simulink model "Snake_Robot_Head_Control"  (R2023a)
settings: Solver=ode23tb  StartTime=0.0  StopTime=2000  FixedStep=0.001  RelTol=1e-3
values from neighbouring files (symbols this model uses):
  cn = 5    [parameters_Robot_control.m]
  ct = 1    [parameters_Robot_control.m]
undefined symbols (not defined in the file or in its folder): X, Y, Z
libraries: nesl_utility x85, sm_lib x49
(part 1 of 3)
settings Model: PacingRate=0.100000  Creator=Bhavik  LastModifiedBy=Bhavik
settings SolverCC: ZeroCrossAlgorithm=Adaptive
settings OptimizationCC: ReuseModelBlockBuffer=off
settings DebuggingCC: UnconnectedInputMsg=warning  UnconnectedOutputMsg=warning  UnconnectedLineMsg=warning
settings ModelReferenceCC: EnableRefExpFcnMdlSchedulingChecks=on
settings RTWCC: DLArmComputeVersion=19.05

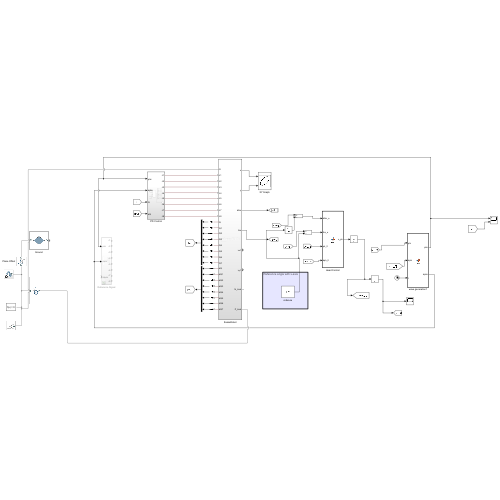
[thumbnail: Simulink's stored preview of the top-level diagram]
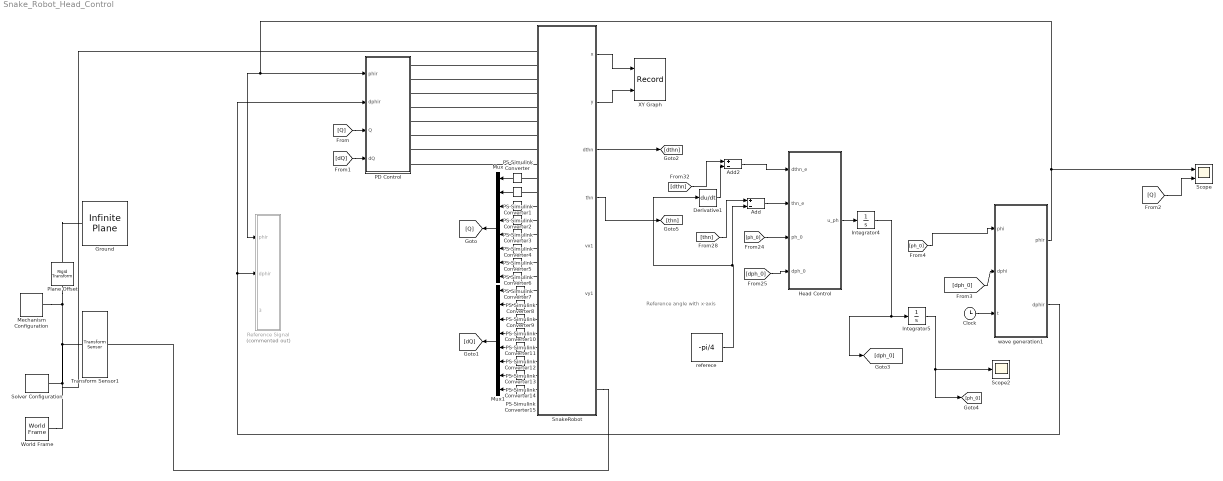
== system Snake_Robot_Head_Control ==
  note: Reference angle with x-axis
  Add : Sum  Inputs=+-
  Add2 : Sum  Inputs=+-
  Clock : Clock
  Derivative1 : Derivative
  Ground : sm_lib/Curves and Surfaces/Infinite Plane  GraphicType=Rectangle  GraphicPlaneWidth=900  GraphicPlaneWidthUnits=m  GraphicPlaneHeight=900  GraphicPlaneHeightUnits=m  GraphicVisPropType=AdvancedVisualProperties  GraphicDiffuseColor=[1 1 1]  GraphicOpacity=1  GraphicSpecularColor=[1 0.4118 0.1608]  GraphicAmbientColor=[0.302 0.7451 0.9333]  GraphicEmissiveColor=[0 1 1]  GraphicShininess=75
  Head Control : MATLAB Function  TreatAsAtomicUnit=on
  Integrator4 : Integrator
  Integrator5 : Integrator
  Mechanism Configuration : sm_lib/Utilities/Mechanism Configuration  UniformGravity=Constant  GravityVector=[0 0 -9.81]  GravityVectorUnits=m/s^2  LinearizationDelta=0.001  JointModeTransitionNonlinearIterations=2
  Mux : Mux  Inputs=8
  Mux1 : Mux  Inputs=8
  PD Control : Subsystem
  PS-Simulink Converter{,1..15} (16 alike) : nesl_utility/PS-Simulink Converter  PhysicalDomain=network_engine_domain  SubClassName=ps_output  LeftPortType=input  RightPortType=output  PseudoPeriodic=off  Frequencies=[]  VectorFormat=inherit  Unit=inherit  AffineConversion=off
  Plane Offset : sm_lib/Frames and Transforms/Rigid Transform  TranslationMethod=StandardAxis  TranslationStandardOffset=50  TranslationStandardOffsetUnits=mm  TranslationStandardAxis=+Z  TranslationCartesianOffset=[0 0 0]  TranslationCartesianOffsetUnits=mm  TranslationROffset=0  TranslationROffsetUnits=m  TranslationZOffset=0  TranslationZOffsetUnits=m  TranslationThetaOffset=0  TranslationThetaOffsetUnits=deg  RotationMethod=None  RotationAngleUnits=deg  RotationStandardAxis=+Z  RotationAngle=0.0  RotationArbitraryAxis=[0 0 1]  FollAlignAxisA=+X  BaseAlignAxisA=+Y  FollAlignAxisB=+Y  BaseAlignAxisB=+Z  RotationSequenceAxes=FollowerAxes  RotationSequence=XYX  RotationSequenceAngles=[0 0 0]  RotationSequenceAnglesUnits=deg  RotationMatrix=[1 0 0; 0 1 0; 0 0 1]  Quaternion=[1 0 0 0]
  Reference Signal : Subsystem  Commented=on
  Scope : Scope  NumInputPorts=2
  Scope2 : Scope
  SnakeRobot : Subsystem
  Solver Configuration : nesl_utility/Solver Configuration  PhysicalDomain=network_engine_domain  SubClassName=solver  LeftPortType=input  RightPortType=generic  Tones=[]  Harmonics=[]  SimulateNoise=off  Profile=off  UseLocalSampling=off  EnableSwitchedLinearOptims=on  FrequencyDomain=off  UseCCode=off  RelTol=0.001  AbsTol=1e-06  MinStep=1e-09  ToWorkspace=off  RevertToSquareIcSolve=off  NumHomotopyIterations=100  PhasorMode=off  PhasorModeNumHarmonics=1  ConsistencySolver=NEWTON_FTOL  IndexReductionMethod=DerivativeReplacement  DoDC=off  ResidualTolerance=1e-09  ConsistencyTolSource=GLOBAL  ConsistencyAbsTol=0.001  ConsistencyRelTol=0.001  ConsistencyTolFactor=0.001  UseLocalSolver=off  LocalSolverChoice=NE_BACKWARD_EULER_ADVANCER  ResolveIndetEquations=on  FunctionEvalNumThread=1  LocalSolverSampleTime=0.001  DoFixedCost=off  MaxNonlinIter=3  MaxModeIter=2  ComputeImpulses=off  ImpulseIterations=2  LinearAlgebra=Sparse  LinearAlgebraNumThread=0  EquationFormulation=NE_TIME_EF  DelaysMemoryBudget=1024  AutomaticFiltering=on  FilteringTimeConstant=0.001  PartitionStorageMethod=AS_NEEDED  PartitionMemoryBudget=1024  PartitionMethod=FAST
  Transform Sensor1 : sm_lib/Frames and Transforms/Transform Sensor  MeasurementFrame=World  RotationSequence=XYX  SenseAngle=off  SenseAxis=off  SenseQ=off  SenseR=off  SenseRotationSequence=off  SenseOmegaX=off  SenseOmegaY=off  SenseOmegaZ=off  SenseQDot=off  SenseRDot=off  SenseRotationSequenceDot=off  SenseAlphaX=off  SenseAlphaY=off  SenseAlphaZ=off  SenseQDDot=off  SenseRDDot=off  SenseX=off  SenseY=off  SenseZ=off  SenseRad=off  SenseAzim=off  SenseDist=off  SenseInc=off  SenseXDot=off  SenseYDot=off  SenseZDot=off  SenseRadDot=off  SenseAzimDot=off  SenseDistDot=off  SenseIncDot=off  SenseXDDot=off  SenseYDDot=off  SenseZDDot=off  SenseRadDDot=off  SenseAzimDDot=off  SenseDistDDot=off  SenseIncDDot=off
  World Frame : sm_lib/Frames and Transforms/World Frame
  XY Graph : Record  FileSettingsInternal="{\"entries\":[{\"content\":{\"excelSettings\":{\"content\":{},\"type\":\"Streamout.ExcelSettings\"}},\"type\":\"Streamout.FileSettingStorage\",\"uuid\":\"\"}],\"packageUris\":[\"http:\\/\\/schema.mathworks.com\\/mf0\\/streamout_blocks\\/R2020a\"],\"version\":\"1.0\"}"  Layout=[1 1]  SignalsInternal="{\"entries\":[{\"content\":{\"signals\":[{\"content\":{\"blockPath\":[],\"dimensions\":[1,1],\"domain\":\"\",\"lineColor\":\"#a2142f\",\"plots\":[1],\"port\":1,\"sid\":[\"\"],\"signalID\":40824,\"signalName\":\"SnakeRobot:1\"},\"type\":\"RecordBlkView.Signal\",\"uuid\":\"\"},{\"content\":{\"blockPath\":[],\"dimensions\":[1,1],\"domain\":\"\",\"lineColor\":\"#139fff\",\"plots\":[1],\"port\":2,\"sid\":[\"\"],\"signalID\":40828,\"signalName\":\"SnakeRobot:2\"},\"type\":\"RecordBlkView.Signal\",\"uuid\":\"\"}]},\"type\":\"RecordBlkView.InputSignals\",\"uuid\":\"\"}],\"packageUris\":[\"http:\\/\\/schema.mathworks.com\\/mf0\\/streamout_blocks\\/R2020a\"],\"version\":\"1.0\"}"  VisualizationBindings="{\"xyplotplugin\":{\"info\":[{\"series\":[{\"bindingParametersList\":[{\"parameter\":\"X-Axis\",\"signalID\":40824,\"signalName\":\"SnakeRobot:1\"},{\"parameter\":\"Y-Axis\",\"signalID\":40828,\"signalName\":\"SnakeRobot:2\"}],\"seriesID\":22525}],\"subplotID\":1}]}}"  CompatibilityTag=XY
  referece : Constant  Value=-pi/4
  wave generation1 : MATLAB Function  TreatAsAtomicUnit=on
  wires:
  SnakeRobot/4(thn) -> [thn]
  SnakeRobot/3(dthn) -> [dthn]
  wave generation1/1(phir) -> PD Control/1(phir), Reference Signal/1(phir), Scope/1
  wave generation1/2(dphir) -> PD Control/2(dphir), Reference Signal/2(dphir)
  PS-Simulink Converter/1 -> Mux/1
  PS-Simulink Converter1/1 -> Mux/2
  PS-Simulink Converter2/1 -> Mux/3
  PS-Simulink Converter3/1 -> Mux/4
  PS-Simulink Converter4/1 -> Mux/5
  PS-Simulink Converter5/1 -> Mux/6
  PS-Simulink Converter6/1 -> Mux/7
  PS-Simulink Converter7/1 -> Mux/8
  PS-Simulink Converter15/1 -> Mux1/8
  PS-Simulink Converter14/1 -> Mux1/7
  PS-Simulink Converter13/1 -> Mux1/6
  PS-Simulink Converter12/1 -> Mux1/5
  PS-Simulink Converter11/1 -> Mux1/4
  PS-Simulink Converter10/1 -> Mux1/3
  PS-Simulink Converter9/1 -> Mux1/2
  PS-Simulink Converter8/1 -> Mux1/1
  Mux/1 -> [Q]
  Mux1/1 -> [dQ]
  [Q] -> PD Control/3(Q)
  [dQ] -> PD Control/4(dQ)
  [dph_0] -> wave generation1/2(dphi)
  SnakeRobot/1(x) -> XY Graph/1
  SnakeRobot/2(y) -> XY Graph/2
  [Q] -> Scope/2
  Integrator5/1 -> [ph_0], Scope2/1
  Clock/1 -> wave generation1/3(t)
  [ph_0] -> Head Control/3(ph_0)
  referece/1 -> Derivative1/1, Add/2
  [dph_0] -> Head Control/4(dph_0)
  Derivative1/1 -> Add2/2
  Head Control/1(u_ph) -> Integrator4/1
  Integrator4/1 -> [dph_0], Integrator5/1
  [thn] -> Add/1
  Add2/1 -> Head Control/1(dthn_e)
  Add/1 -> Head Control/2(thn_e)
  [dthn] -> Add2/1
  [ph_0] -> wave generation1/1(phi)
  connections:
  Plane Offset/LConn1 -- Ground/LConn1
  Transform Sensor1/LConn1 -- SnakeRobot/LConn1 -- World Frame/RConn1 -- Solver Configuration/RConn1 -- Plane Offset/RConn1 -- Mechanism Configuration/RConn1
  SnakeRobot/RConn2 -- Transform Sensor1/RConn1
  SnakeRobot/LConn10 -- PS-Simulink Converter/LConn1
  SnakeRobot/LConn11 -- PS-Simulink Converter1/LConn1
  SnakeRobot/LConn12 -- PS-Simulink Converter2/LConn1
  SnakeRobot/LConn13 -- PS-Simulink Converter3/LConn1
  SnakeRobot/LConn14 -- PS-Simulink Converter4/LConn1
  SnakeRobot/LConn15 -- PS-Simulink Converter5/LConn1
  SnakeRobot/LConn16 -- PS-Simulink Converter6/LConn1
  SnakeRobot/LConn17 -- PS-Simulink Converter7/LConn1
  SnakeRobot/LConn25 -- PS-Simulink Converter15/LConn1
  SnakeRobot/LConn24 -- PS-Simulink Converter14/LConn1
  SnakeRobot/LConn22 -- PS-Simulink Converter12/LConn1
  SnakeRobot/LConn21 -- PS-Simulink Converter11/LConn1
  SnakeRobot/LConn19 -- PS-Simulink Converter9/LConn1
  SnakeRobot/LConn20 -- PS-Simulink Converter10/LConn1
  SnakeRobot/LConn23 -- PS-Simulink Converter13/LConn1
  SnakeRobot/LConn18 -- PS-Simulink Converter8/LConn1
  SnakeRobot/LConn9 -- PD Control/RConn8
  SnakeRobot/LConn8 -- PD Control/RConn7
  SnakeRobot/LConn7 -- PD Control/RConn6
  SnakeRobot/LConn6 -- PD Control/RConn5
  SnakeRobot/LConn5 -- PD Control/RConn4
  SnakeRobot/LConn4 -- PD Control/RConn3
  SnakeRobot/LConn3 -- PD Control/RConn2
  SnakeRobot/LConn2 -- PD Control/RConn1

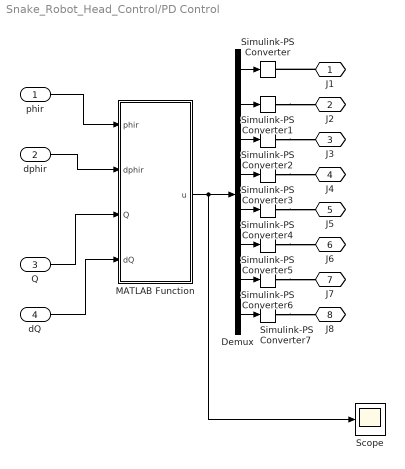
== system Snake_Robot_Head_Control/PD Control ==
  phir : Inport
  dphir : Inport  Port=2
  Q : Inport  Port=3
  dQ : Inport  Port=4
  Demux : Demux  Outputs=8
  MATLAB Function : MATLAB Function  TreatAsAtomicUnit=on
  Scope : Scope
  Simulink-PS Converter{,1..7} (8 alike) : nesl_utility/Simulink-PS Converter  PhysicalDomain=network_engine_domain  SubClassName=ps_input  LeftPortType=input  RightPortType=output  PseudoPeriodic=off  Frequencies=[]  NoiseDistribution=none  NoiseParameters=[]  Unit=1  AffineConversion=off  FilteringAndDerivatives=provide  SimscapeFilterOrder=1  InputFilterTimeConstant=0.001  UdotUserProvided=0
  J1 : PMIOPort  Side=Right
  J2 : PMIOPort  Port=2  Side=Right
  J3 : PMIOPort  Port=3  Side=Right
  J4 : PMIOPort  Port=4  Side=Right
  J5 : PMIOPort  Port=5  Side=Right
  J6 : PMIOPort  Port=6  Side=Right
  J7 : PMIOPort  Port=7  Side=Right
  J8 : PMIOPort  Port=8  Side=Right
  wires:
  phir/1 -> MATLAB Function/1(phir)
  dphir/1 -> MATLAB Function/2(dphir)
  Q/1 -> MATLAB Function/3(Q)
  dQ/1 -> MATLAB Function/4(dQ)
  MATLAB Function/1(u) -> Demux/1, Scope/1
  Demux/1 -> Simulink-PS Converter/1
  Demux/2 -> Simulink-PS Converter1/1
  Demux/3 -> Simulink-PS Converter2/1
  Demux/4 -> Simulink-PS Converter3/1
  Demux/5 -> Simulink-PS Converter4/1
  Demux/6 -> Simulink-PS Converter5/1
  Demux/7 -> Simulink-PS Converter6/1
  Demux/8 -> Simulink-PS Converter7/1
  connections:
  J1/RConn1 -- Simulink-PS Converter/RConn1
  Simulink-PS Converter1/RConn1 -- J2/RConn1
  Simulink-PS Converter2/RConn1 -- J3/RConn1
  Simulink-PS Converter3/RConn1 -- J4/RConn1
  Simulink-PS Converter4/RConn1 -- J5/RConn1
  Simulink-PS Converter5/RConn1 -- J6/RConn1
  Simulink-PS Converter6/RConn1 -- J7/RConn1
  Simulink-PS Converter7/RConn1 -- J8/RConn1

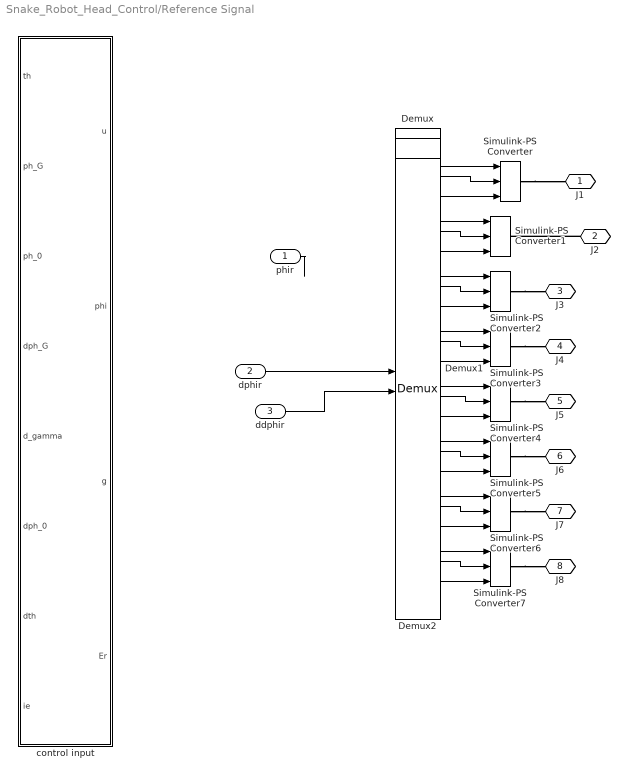
== system Snake_Robot_Head_Control/Reference Signal ==
  phir : Inport
  dphir : Inport  Port=2
  ddphir : Inport  Port=3
  Demux : Demux  Outputs=8
  Demux1 : Demux  Outputs=8
  Demux2 : Demux  Outputs=8
  Simulink-PS Converter{,1..7} (8 alike) : nesl_utility/Simulink-PS Converter  PhysicalDomain=network_engine_domain  SubClassName=ps_input  LeftPortType=input  RightPortType=output  PseudoPeriodic=off  Frequencies=[]  NoiseDistribution=none  NoiseParameters=[]  Unit=rad  AffineConversion=off  FilteringAndDerivatives=provide  SimscapeFilterOrder=1  InputFilterTimeConstant=0.001  UdotUserProvided=2
  control input : MATLAB Function  TreatAsAtomicUnit=on
  J1 : PMIOPort  Side=Right
  J2 : PMIOPort  Port=2  Side=Right
  J3 : PMIOPort  Port=3  Side=Right
  J4 : PMIOPort  Port=4  Side=Right
  J5 : PMIOPort  Port=5  Side=Right
  J6 : PMIOPort  Port=6  Side=Right
  J7 : PMIOPort  Port=7  Side=Right
  J8 : PMIOPort  Port=8  Side=Right
  wires:
  phir/1 -> ?
  Demux/1 -> Simulink-PS Converter/1
  dphir/1 -> Demux1/1
  ddphir/1 -> Demux2/1
  Demux1/1 -> Simulink-PS Converter/2
  Demux2/1 -> Simulink-PS Converter/3
  Demux/2 -> Simulink-PS Converter1/1
  Demux2/2 -> Simulink-PS Converter1/3
  Demux1/2 -> Simulink-PS Converter1/2
  Demux/3 -> Simulink-PS Converter2/1
  Demux2/3 -> Simulink-PS Converter2/3
  Demux1/3 -> Simulink-PS Converter2/2
  Demux/4 -> Simulink-PS Converter3/1
  Demux2/4 -> Simulink-PS Converter3/3
  Demux1/4 -> Simulink-PS Converter3/2
  Demux/5 -> Simulink-PS Converter4/1
  Demux2/5 -> Simulink-PS Converter4/3
  Demux1/5 -> Simulink-PS Converter4/2
  Demux/6 -> Simulink-PS Converter5/1
  Demux2/6 -> Simulink-PS Converter5/3
  Demux1/6 -> Simulink-PS Converter5/2
  Demux/7 -> Simulink-PS Converter6/1
  Demux2/7 -> Simulink-PS Converter6/3
  Demux1/7 -> Simulink-PS Converter6/2
  Demux/8 -> Simulink-PS Converter7/1
  Demux2/8 -> Simulink-PS Converter7/3
  Demux1/8 -> Simulink-PS Converter7/2
  connections:
  Simulink-PS Converter/RConn1 -- J1/RConn1
  J2/RConn1 -- Simulink-PS Converter1/RConn1
  Simulink-PS Converter2/RConn1 -- J3/RConn1
  Simulink-PS Converter3/RConn1 -- J4/RConn1
  Simulink-PS Converter4/RConn1 -- J5/RConn1
  Simulink-PS Converter5/RConn1 -- J6/RConn1
  Simulink-PS Converter6/RConn1 -- J7/RConn1
  Simulink-PS Converter7/RConn1 -- J8/RConn1

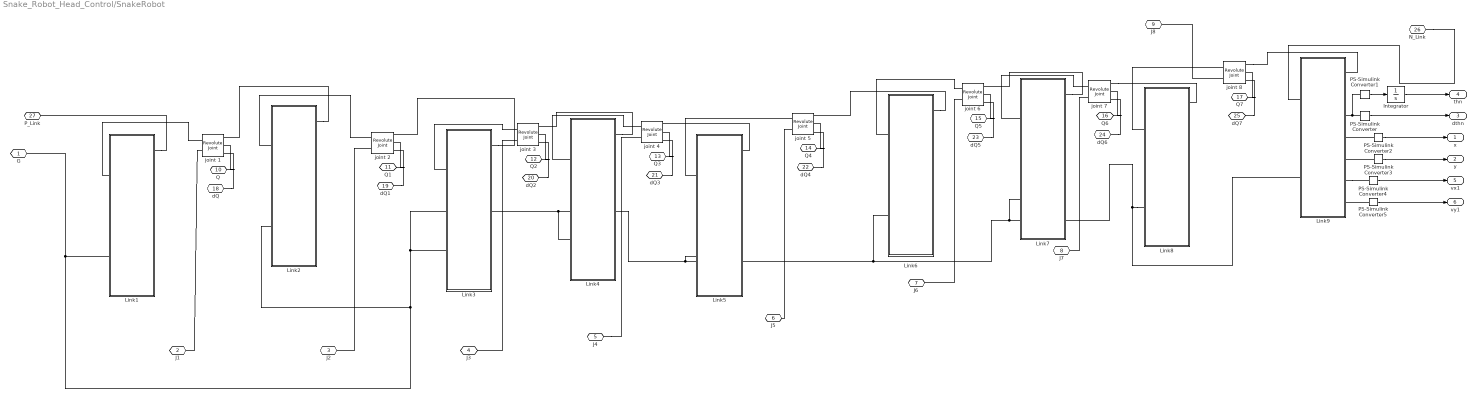
== system Snake_Robot_Head_Control/SnakeRobot ==
  Integrator : Integrator
  Link1 : Subsystem
  Link2 : Subsystem
  Link3 : Subsystem
  Link4 : Subsystem
  Link5 : Subsystem
  Link6 : Subsystem
  Link7 : Subsystem
  Link8 : Subsystem
  Link9 : Subsystem
  PS-Simulink Converter{,1..5} (6 alike) : nesl_utility/PS-Simulink Converter  PhysicalDomain=network_engine_domain  SubClassName=ps_output  LeftPortType=input  RightPortType=output  PseudoPeriodic=off  Frequencies=[]  VectorFormat=inherit  Unit=inherit  AffineConversion=off
  joint {1..8} (8 alike) : sm_lib/Joints/Revolute Joint  JointMode=Normal  SenseConstraintForce=off  SenseConstraintForceX=off  SenseConstraintForceY=off  SenseConstraintForceZ=off  SenseConstraintTorque=off  SenseConstraintTorqueX=off  SenseConstraintTorqueY=off  SenseConstraintTorqueZ=off  SenseTotalForce=off  SenseTotalForceX=off  SenseTotalForceY=off  SenseTotalForceZ=off  SenseTotalTorque=off  SenseTotalTorqueX=off  SenseTotalTorqueY=off  SenseTotalTorqueZ=off  CompositeWrenchDir=FollowerOnBase  CompositeWrenchFrame=BaseFrame  EquilibriumPosition=0  EquilibriumPositionUnits=deg  SpringStiffness=internal_stiffness  SpringStiffnessUnits=N*m/deg  DampingCoefficient=internal_damping  DampingCoefficientUnits=N*m/(deg/s)  TorqueActuationMode=InputTorque  MotionActuationMode=ComputedMotion  SensePosition=on  SenseVelocity=on  SenseAcceleration=off  SenseTorqueForce=off  SenseLowerLimitTorqueForce=off  SenseUpperLimitTorqueForce=off  LowerLimitSpecify=on  LowerLimitBound=-90  LowerLimitBoundUnits=deg  LowerLimitStiffness=spring_stiffness  LowerLimitStiffnessUnits=N*m/deg  LowerLimitDamping=joint_damp  LowerLimitDampingUnits=N*m/(deg/s)  LowerLimitTransitionRegionWidth=0.1  LowerLimitTransitionRegionWidthUnits=deg  UpperLimitSpecify=on  UpperLimitBound=90  UpperLimitBoundUnits=deg  UpperLimitStiffness=spring_stiffness  UpperLimitStiffnessUnits=N*m/deg  UpperLimitDamping=joint_damp  UpperLimitDampingUnits=N*m/(deg/s)  UpperLimitTransitionRegionWidth=0.1  UpperLimitTransitionRegionWidthUnits=deg  PositionTargetSpecify=off  PositionTargetPriority=High  PositionTargetValue=0  PositionTargetValueUnits=deg  VelocityTargetSpecify=off  VelocityTargetPriority=High  VelocityTargetValue=0  VelocityTargetValueUnits=deg/s
  G : PMIOPort  Side=Left
  J1 : PMIOPort  Port=2  Side=Left
  J2 : PMIOPort  Port=3  Side=Left
  J3 : PMIOPort  Port=4  Side=Left
  J4 : PMIOPort  Port=5  Side=Left
  J5 : PMIOPort  Port=6  Side=Left
  J6 : PMIOPort  Port=7  Side=Left
  J7 : PMIOPort  Port=8  Side=Left
  J8 : PMIOPort  Port=9  Side=Left
  Q : PMIOPort  Port=10  Side=Left
  Q1 : PMIOPort  Port=11  Side=Left
  Q2 : PMIOPort  Port=12  Side=Left
  Q3 : PMIOPort  Port=13  Side=Left
  Q4 : PMIOPort  Port=14  Side=Left
  Q5 : PMIOPort  Port=15  Side=Left
  Q6 : PMIOPort  Port=16  Side=Left
  Q7 : PMIOPort  Port=17  Side=Left
  dQ : PMIOPort  Port=18  Side=Left
  dQ1 : PMIOPort  Port=19  Side=Left
  dQ2 : PMIOPort  Port=20  Side=Left
  dQ3 : PMIOPort  Port=21  Side=Left
  dQ4 : PMIOPort  Port=22  Side=Left
  dQ5 : PMIOPort  Port=23  Side=Left
  dQ6 : PMIOPort  Port=24  Side=Left
  dQ7 : PMIOPort  Port=25  Side=Left
  N_Link : PMIOPort  Port=26  Side=Right
  P_Link : PMIOPort  Port=27  Side=Right
  x : Outport
  y : Outport  Port=2
  dthn : Outport  Port=3
  thn : Outport  Port=4
  vx1 : Outport  Port=5
  vy1 : Outport  Port=6
  wires:
  PS-Simulink Converter1/1 -> Integrator/1
  PS-Simulink Converter/1 -> dthn/1
  PS-Simulink Converter3/1 -> y/1
  PS-Simulink Converter5/1 -> vy1/1
  PS-Simulink Converter4/1 -> vx1/1
  PS-Simulink Converter2/1 -> x/1
  Integrator/1 -> thn/1
  connections:
  Link8/LConn2 -- Link9/LConn2 -- Link7/LConn2 -- Link6/LConn2 -- Link5/LConn2 -- Link4/LConn2 -- Link3/LConn2 -- Link2/LConn2 -- G/RConn1 -- Link1/LConn2
  Q7/RConn1 -- joint 8/RConn2
  dQ7/RConn1 -- joint 8/RConn3
  Link2/LConn1 -- joint 2/LConn1
  Link6/LConn1 -- joint 6/LConn1
  Link5/LConn1 -- joint 5/LConn1
  Q2/RConn1 -- joint 3/RConn2
  Link9/RConn6 -- PS-Simulink Converter4/LConn1
  dQ2/RConn1 -- joint 3/RConn3
  J4/RConn1 -- joint 4/LConn2
  dQ5/RConn1 -- joint 6/RConn3
  PS-Simulink Converter2/LConn1 -- Link9/RConn4
  dQ/RConn1 -- joint 1/RConn3
  Q3/RConn1 -- joint 4/RConn2
  Link9/RConn3 -- PS-Simulink Converter1/LConn1 -- PS-Simulink Converter/LConn1
  Link3/LConn1 -- joint 3/LConn1
  joint 8/LConn2 -- J8/RConn1
  joint 6/LConn2 -- J6/RConn1
  dQ1/RConn1 -- joint 2/RConn3
  N_Link/RConn1 -- Link9/LConn1
  Link3/RConn1 -- joint 2/RConn1
  Q1/RConn1 -- joint 2/RConn2
  dQ4/RConn1 -- joint 5/RConn3
  joint 3/LConn2 -- J3/RConn1
  Q5/RConn1 -- joint 6/RConn2
  joint 8/RConn1 -- Link9/RConn1
  Link4/RConn1 -- joint 3/RConn1
  joint 5/LConn2 -- J5/RConn1
  Link1/LConn1 -- joint 1/LConn1
  Link7/LConn1 -- joint 7/LConn1
  Q6/RConn1 -- joint 7/RConn2
  J1/RConn1 -- joint 1/LConn2
  dQ3/RConn1 -- joint 4/RConn3
  Link5/RConn1 -- joint 4/RConn1
  Q4/RConn1 -- joint 5/RConn2
  Link6/RConn1 -- joint 5/RConn1
  joint 8/LConn1 -- Link8/LConn1
  joint 7/LConn2 -- J7/RConn1
  PS-Simulink Converter3/LConn1 -- Link9/RConn5
  Link2/RConn1 -- joint 1/RConn1
  Q/RConn1 -- joint 1/RConn2
  dQ6/RConn1 -- joint 7/RConn3
  Link7/RConn1 -- joint 6/RConn1
  joint 7/RConn1 -- Link8/RConn1
  joint 2/LConn2 -- J2/RConn1
  Link4/LConn1 -- joint 4/LConn1
  PS-Simulink Converter5/LConn1 -- Link9/RConn7
  Link1/RConn1 -- P_Link/RConn1

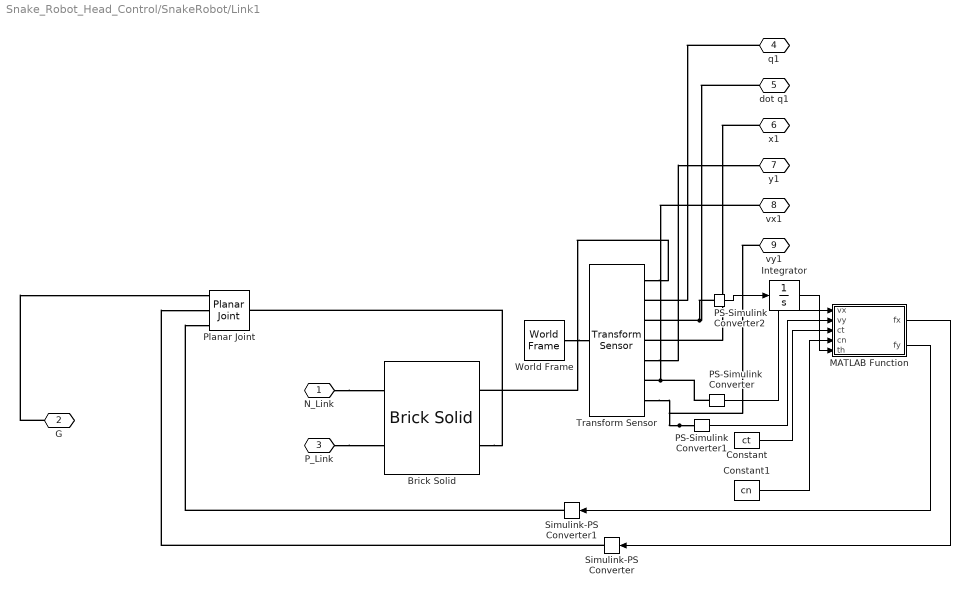
== system Snake_Robot_Head_Control/SnakeRobot/Link1 ==
  Brick Solid : sm_lib/Body Elements/Brick Solid  GraphicAmbientColor=[0.15 0.15 0.15 1.0]  BasedOnType=Mass  BrickDimensions=[180 80 80]  BrickDimensionsUnits=mm  CenterOfMass=[0 0 0]  CenterOfMassUnits=m  GraphicDiffuseColor=[0.5 0.5 0.5]  Density=1000  DensityUnits=kg/m^3  DoExposeReferenceFrame=on  GraphicEmissiveColor=[0.0 0.0 0.0 1.0]  ExportEntireGeometry=off  SerializedFrames=<Frames><Frame><Id>Frame1</Id><Value><Name>nextlink</Name><Origin><Source>GeometricFeature</Source><FeatureName>+x surface</FeatureName></Origin><PrimaryAxis><DefinedDirection>+Z</DefinedDirection><Source>ReferenceFrame</Source><SourceDirection>+Z</SourceDirection><FeatureName></FeatureName></PrimaryAxis><SecondaryAxis><DefinedDirection>+X</DefinedDirection><Source>ReferenceFrame</Source><SourceDirection>+X</SourceDirection><FeatureName></FeatureName></SecondaryAxis></Value></Frame><Frame><Id>Frame2</Id><Value><Name>P_link</Name><Origin><Source>GeometricFeature</Source><FeatureName>-x surface</FeatureName></Origin><PrimaryAxis><DefinedDirection>+Z</DefinedDirection><Source>ReferenceFrame</Source><SourceDirection>+Z</SourceDirection><FeatureName></FeatureName></PrimaryAxis><SecondaryAxis><DefinedDirection>+X</DefinedDirection><Source>ReferenceFrame</Source><SourceDirection>+X</SourceDirection><FeatureName></FeatureName></SecondaryAxis></Value></Frame><Frame><Id>Frame3</Id><Value><Name>F3</Name><Origin><Source>CenterOfMassFrame</Source><FeatureName></FeatureName></Origin><PrimaryAxis><DefinedDirection>+Z</DefinedDirection><Source>ReferenceFrame</Source><SourceDirection>+Z</SourceDirection><FeatureName></FeatureName></PrimaryAxis><SecondaryAxis><DefinedDirection>+X</DefinedDirection><Source>ReferenceFrame</Source><SourceDirection>+X</SourceDirection><FeatureName></FeatureName></SecondaryAxis></Value></Frame></Frames>  MarkerShape=Sphere  MarkerSize=10  GraphicType=FromGeometry  InertiaType=CalculateFromGeometry  Mass=0.9047  MassUnits=kg  MomentsOfInertia=[1 1 1]  MomentsOfInertiaUnits=kg*m^2  GraphicOpacity=1.0  ProductsOfInertia=[0 0 0]  ProductsOfInertiaUnits=kg*m^2  GraphicShininess=75  GraphicSpecularColor=[0.5 0.5 0.5 1.0]  GraphicVisPropType=SimpleVisualProperties
  Constant : Constant  Value=ct
  Constant1 : Constant  Value=cn
  Integrator : Integrator
  MATLAB Function : MATLAB Function  TreatAsAtomicUnit=on
  PS-Simulink Converter : nesl_utility/PS-Simulink Converter  PhysicalDomain=network_engine_domain  SubClassName=ps_output  LeftPortType=input  RightPortType=output  PseudoPeriodic=off  Frequencies=[]  VectorFormat=inherit  Unit=inherit  AffineConversion=off
  PS-Simulink Converter1 : nesl_utility/PS-Simulink Converter  PhysicalDomain=network_engine_domain  SubClassName=ps_output  LeftPortType=input  RightPortType=output  PseudoPeriodic=off  Frequencies=[]  VectorFormat=inherit  Unit=inherit  AffineConversion=off
  PS-Simulink Converter2 : nesl_utility/PS-Simulink Converter  PhysicalDomain=network_engine_domain  SubClassName=ps_output  LeftPortType=input  RightPortType=output  PseudoPeriodic=off  Frequencies=[]  VectorFormat=inherit  Unit=inherit  AffineConversion=off
  Planar Joint : sm_lib/Joints/Planar Joint  JointMode=Normal  SenseConstraintForce=off  SenseConstraintForceX=off  SenseConstraintForceY=off  SenseConstraintForceZ=off  SenseConstraintTorque=off  SenseConstraintTorqueX=off  SenseConstraintTorqueY=off  SenseConstraintTorqueZ=off  SenseTotalForce=off  SenseTotalForceX=off  SenseTotalForceY=off  SenseTotalForceZ=off  SenseTotalTorque=off  SenseTotalTorqueX=off  SenseTotalTorqueY=off  SenseTotalTorqueZ=off  CompositeWrenchDir=FollowerOnBase  CompositeWrenchFrame=BaseFrame  PxEquilibriumPosition=0  PxEquilibriumPositionUnits=m  PxSpringStiffness=0  PxSpringStiffnessUnits=N/m  PxDampingCoefficient=0  PxDampingCoefficientUnits=N/(m/s)  PxTorqueActuationMode=InputTorque  PxMotionActuationMode=ComputedMotion  PxSensePosition=off  PxSenseVelocity=off  PxSenseAcceleration=off  PxSenseTorqueForce=off  PxSenseLowerLimitTorqueForce=off  PxSenseUpperLimitTorqueForce=off  PxLowerLimitSpecify=off  PxLowerLimitBound=-1  PxLowerLimitBoundUnits=m  PxLowerLimitStiffness=1e6  PxLowerLimitStiffnessUnits=N/m  PxLowerLimitDamping=1e3  PxLowerLimitDampingUnits=N/(m/s)  PxLowerLimitTransitionRegionWidth=1e-4  PxLowerLimitTransitionRegionWidthUnits=m  PxUpperLimitSpecify=off  PxUpperLimitBound=1  PxUpperLimitBoundUnits=m  PxUpperLimitStiffness=1e6  PxUpperLimitStiffnessUnits=N/m  PxUpperLimitDamping=1e3  PxUpperLimitDampingUnits=N/(m/s)  PxUpperLimitTransitionRegionWidth=1e-4  PxUpperLimitTransitionRegionWidthUnits=m  PxPositionTargetSpecify=off  PxPositionTargetPriority=High  PxPositionTargetValue=0  PxPositionTargetValueUnits=m  PxVelocityTargetSpecify=off  PxVelocityTargetPriority=High  PxVelocityTargetValue=0  PxVelocityTargetValueUnits=m/s  PyEquilibriumPosition=0  PyEquilibriumPositionUnits=m  PySpringStiffness=0  PySpringStiffnessUnits=N/m  PyDampingCoefficient=0  PyDampingCoefficientUnits=N/(m/s)  PyTorqueActuationMode=InputTorque  PyMotionActuationMode=ComputedMotion  PySensePosition=off  PySenseVelocity=off  PySenseAcceleration=off  PySenseTorqueForce=off  PySenseLowerLimitTorqueForce=off  PySenseUpperLimitTorqueForce=off  PyLowerLimitSpecify=off  PyLowerLimitBound=-1  PyLowerLimitBoundUnits=m  PyLowerLimitStiffness=1e6  PyLowerLimitStiffnessUnits=N/m  PyLowerLimitDamping=1e3  PyLowerLimitDampingUnits=N/(m/s)  PyLowerLimitTransitionRegionWidth=1e-4  PyLowerLimitTransitionRegionWidthUnits=m  PyUpperLimitSpecify=off  PyUpperLimitBound=1  PyUpperLimitBoundUnits=m  PyUpperLimitStiffness=1e6  PyUpperLimitStiffnessUnits=N/m  PyUpperLimitDamping=1e3  PyUpperLimitDampingUnits=N/(m/s)  PyUpperLimitTransitionRegionWidth=1e-4  PyUpperLimitTransitionRegionWidthUnits=m  PyPositionTargetSpecify=off  PyPositionTargetPriority=High  PyPositionTargetValue=0  PyPositionTargetValueUnits=m  PyVelocityTargetSpecify=off  PyVelocityTargetPriority=High  PyVelocityTargetValue=0  PyVelocityTargetValueUnits=m/s  RzEquilibriumPosition=0  RzEquilibriumPositionUnits=deg  RzSpringStiffness=0  RzSpringStiffnessUnits=N*m/deg  RzDampingCoefficient=0  RzDampingCoefficientUnits=N*m/(deg/s)  RzTorqueActuationMode=NoTorque  RzMotionActuationMode=ComputedMotion  RzSensePosition=off  RzSenseVelocity=off  RzSenseAcceleration=off  RzSenseTorqueForce=off  RzSenseLowerLimitTorqueForce=off  RzSenseUpperLimitTorqueForce=off  RzLowerLimitSpecify=off  RzLowerLimitBound=-90  RzLowerLimitBoundUnits=deg  RzLowerLimitStiffness=1e4  RzLowerLimitStiffnessUnits=N*m/deg  RzLowerLimitDamping=10  RzLowerLimitDampingUnits=N*m/(deg/s)  RzLowerLimitTransitionRegionWidth=0.1  RzLowerLimitTransitionRegionWidthUnits=deg  RzUpperLimitSpecify=off  RzUpperLimitBound=90  RzUpperLimitBoundUnits=deg  RzUpperLimitStiffness=1e4  RzUpperLimitStiffnessUnits=N*m/deg  RzUpperLimitDamping=10  RzUpperLimitDampingUnits=N*m/(deg/s)  RzUpperLimitTransitionRegionWidth=0.1  RzUpperLimitTransitionRegionWidthUnits=deg  RzPositionTargetSpecify=off  RzPositionTargetPriority=High  RzPositionTargetValue=0  RzPositionTargetValueUnits=deg  RzVelocityTargetSpecify=off  RzVelocityTargetPriority=High  RzVelocityTargetValue=0  RzVelocityTargetValueUnits=deg/s
  Simulink-PS Converter : nesl_utility/Simulink-PS Converter  PhysicalDomain=network_engine_domain  SubClassName=ps_input  LeftPortType=input  RightPortType=output  PseudoPeriodic=off  Frequencies=[]  NoiseDistribution=none  NoiseParameters=[]  Unit=1  AffineConversion=off  FilteringAndDerivatives=provide  SimscapeFilterOrder=1  InputFilterTimeConstant=0.001  UdotUserProvided=0
  Simulink-PS Converter1 : nesl_utility/Simulink-PS Converter  PhysicalDomain=network_engine_domain  SubClassName=ps_input  LeftPortType=input  RightPortType=output  PseudoPeriodic=off  Frequencies=[]  NoiseDistribution=none  NoiseParameters=[]  Unit=1  AffineConversion=off  FilteringAndDerivatives=provide  SimscapeFilterOrder=1  InputFilterTimeConstant=0.001  UdotUserProvided=0
  Transform Sensor : sm_lib/Frames and Transforms/Transform Sensor  MeasurementFrame=World  RotationSequence=XYX  SenseAngle=on  SenseAxis=off  SenseQ=off  SenseR=off  SenseRotationSequence=off  SenseOmegaX=off  SenseOmegaY=off  SenseOmegaZ=on  SenseQDot=off  SenseRDot=off  SenseRotationSequenceDot=off  SenseAlphaX=off  SenseAlphaY=off  SenseAlphaZ=off  SenseQDDot=off  SenseRDDot=off  SenseX=on  SenseY=on  SenseZ=off  SenseRad=off  SenseAzim=off  SenseDist=off  SenseInc=off  SenseXDot=on  SenseYDot=on  SenseZDot=off  SenseRadDot=off  SenseAzimDot=off  SenseDistDot=off  SenseIncDot=off  SenseXDDot=off  SenseYDDot=off  SenseZDDot=off  SenseRadDDot=off  SenseAzimDDot=off  SenseDistDDot=off  SenseIncDDot=off
  World Frame : sm_lib/Frames and Transforms/World Frame
  N_Link : PMIOPort  Side=Left
  G : PMIOPort  Port=2  Side=Left
  P_Link : PMIOPort  Port=3  Side=Right
  q1 : PMIOPort  Port=4  Side=Right
  dot q1 : PMIOPort  Port=5  Side=Right
  x1 : PMIOPort  Port=6  Side=Right
  y1 : PMIOPort  Port=7  Side=Right
  vx1 : PMIOPort  Port=8  Side=Right
  vy1 : PMIOPort  Port=9  Side=Right
  wires:
  PS-Simulink Converter2/1 -> Integrator/1
  Constant1/1 -> MATLAB Function/4(cn)
  Constant/1 -> MATLAB Function/3(ct)
  Integrator/1 -> MATLAB Function/5(th)
  PS-Simulink Converter/1 -> MATLAB Function/1(vx)
  PS-Simulink Converter1/1 -> MATLAB Function/2(vy)
  MATLAB Function/2(fy) -> Simulink-PS Converter1/1
  MATLAB Function/1(fx) -> Simulink-PS Converter/1
  connections:
  dot q1/RConn1 -- Transform Sensor/RConn3 -- PS-Simulink Converter2/LConn1
  PS-Simulink Converter1/LConn1 -- Transform Sensor/RConn7 -- vy1/RConn1
  vx1/RConn1 -- Transform Sensor/RConn6 -- PS-Simulink Converter/LConn1
  Transform Sensor/RConn5 -- y1/RConn1
  Transform Sensor/RConn1 -- Brick Solid/RConn1
  x1/RConn1 -- Transform Sensor/RConn4
  P_Link/RConn1 -- Brick Solid/LConn2
  N_Link/RConn1 -- Brick Solid/LConn1
  World Frame/RConn1 -- Transform Sensor/LConn1
  q1/RConn1 -- Transform Sensor/RConn2
  G/RConn1 -- Planar Joint/LConn1
  Simulink-PS Converter1/RConn1 -- Planar Joint/LConn3
  Simulink-PS Converter/RConn1 -- Planar Joint/LConn2
  Brick Solid/RConn2 -- Planar Joint/RConn1

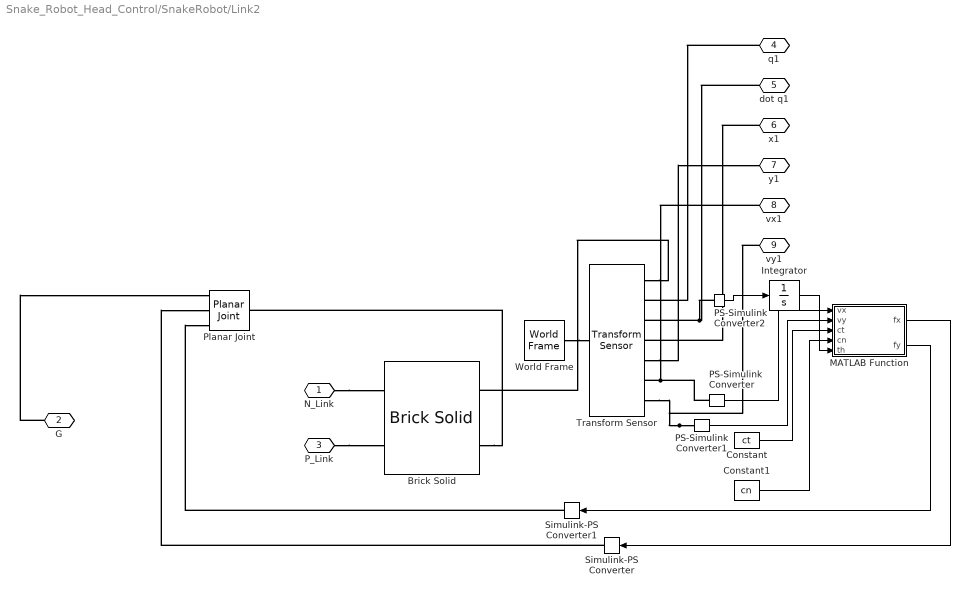
== system Snake_Robot_Head_Control/SnakeRobot/Link2 ==
  Brick Solid : sm_lib/Body Elements/Brick Solid  GraphicAmbientColor=[0.15 0.15 0.15 1.0]  BasedOnType=Mass  BrickDimensions=[180 80 80]  BrickDimensionsUnits=mm  CenterOfMass=[0 0 0]  CenterOfMassUnits=m  GraphicDiffuseColor=[0.5 0.5 0.5]  Density=1000  DensityUnits=kg/m^3  DoExposeReferenceFrame=on  GraphicEmissiveColor=[0.0 0.0 0.0 1.0]  ExportEntireGeometry=off  SerializedFrames=<Frames><Frame><Id>Frame1</Id><Value><Name>nextlink</Name><Origin><Source>GeometricFeature</Source><FeatureName>+x surface</FeatureName></Origin><PrimaryAxis><DefinedDirection>+Z</DefinedDirection><Source>ReferenceFrame</Source><SourceDirection>+Z</SourceDirection><FeatureName></FeatureName></PrimaryAxis><SecondaryAxis><DefinedDirection>+X</DefinedDirection><Source>ReferenceFrame</Source><SourceDirection>+X</SourceDirection><FeatureName></FeatureName></SecondaryAxis></Value></Frame><Frame><Id>Frame2</Id><Value><Name>P_link</Name><Origin><Source>GeometricFeature</Source><FeatureName>-x surface</FeatureName></Origin><PrimaryAxis><DefinedDirection>+Z</DefinedDirection><Source>ReferenceFrame</Source><SourceDirection>+Z</SourceDirection><FeatureName></FeatureName></PrimaryAxis><SecondaryAxis><DefinedDirection>+X</DefinedDirection><Source>ReferenceFrame</Source><SourceDirection>+X</SourceDirection><FeatureName></FeatureName></SecondaryAxis></Value></Frame><Frame><Id>Frame3</Id><Value><Name>F3</Name><Origin><Source>CenterOfMassFrame</Source><FeatureName></FeatureName></Origin><PrimaryAxis><DefinedDirection>+Z</DefinedDirection><Source>ReferenceFrame</Source><SourceDirection>+Z</SourceDirection><FeatureName></FeatureName></PrimaryAxis><SecondaryAxis><DefinedDirection>+X</DefinedDirection><Source>ReferenceFrame</Source><SourceDirection>+X</SourceDirection><FeatureName></FeatureName></SecondaryAxis></Value></Frame></Frames>  MarkerShape=Sphere  MarkerSize=10  GraphicType=FromGeometry  InertiaType=CalculateFromGeometry  Mass=0.9047  MassUnits=kg  MomentsOfInertia=[1 1 1]  MomentsOfInertiaUnits=kg*m^2  GraphicOpacity=1.0  ProductsOfInertia=[0 0 0]  ProductsOfInertiaUnits=kg*m^2  GraphicShininess=75  GraphicSpecularColor=[0.5 0.5 0.5 1.0]  GraphicVisPropType=SimpleVisualProperties
  Constant : Constant  Value=ct
  Constant1 : Constant  Value=cn
  Integrator : Integrator
  MATLAB Function : MATLAB Function  TreatAsAtomicUnit=on
  PS-Simulink Converter : nesl_utility/PS-Simulink Converter  PhysicalDomain=network_engine_domain  SubClassName=ps_output  LeftPortType=input  RightPortType=output  PseudoPeriodic=off  Frequencies=[]  VectorFormat=inherit  Unit=inherit  AffineConversion=off
  PS-Simulink Converter1 : nesl_utility/PS-Simulink Converter  PhysicalDomain=network_engine_domain  SubClassName=ps_output  LeftPortType=input  RightPortType=output  PseudoPeriodic=off  Frequencies=[]  VectorFormat=inherit  Unit=inherit  AffineConversion=off
  PS-Simulink Converter2 : nesl_utility/PS-Simulink Converter  PhysicalDomain=network_engine_domain  SubClassName=ps_output  LeftPortType=input  RightPortType=output  PseudoPeriodic=off  Frequencies=[]  VectorFormat=inherit  Unit=inherit  AffineConversion=off
  Planar Joint : sm_lib/Joints/Planar Joint  JointMode=Normal  SenseConstraintForce=off  SenseConstraintForceX=off  SenseConstraintForceY=off  SenseConstraintForceZ=off  SenseConstraintTorque=off  SenseConstraintTorqueX=off  SenseConstraintTorqueY=off  SenseConstraintTorqueZ=off  SenseTotalForce=off  SenseTotalForceX=off  SenseTotalForceY=off  SenseTotalForceZ=off  SenseTotalTorque=off  SenseTotalTorqueX=off  SenseTotalTorqueY=off  SenseTotalTorqueZ=off  CompositeWrenchDir=FollowerOnBase  CompositeWrenchFrame=BaseFrame  PxEquilibriumPosition=0  PxEquilibriumPositionUnits=m  PxSpringStiffness=0  PxSpringStiffnessUnits=N/m  PxDampingCoefficient=0  PxDampingCoefficientUnits=N/(m/s)  PxTorqueActuationMode=InputTorque  PxMotionActuationMode=ComputedMotion  PxSensePosition=off  PxSenseVelocity=off  PxSenseAcceleration=off  PxSenseTorqueForce=off  PxSenseLowerLimitTorqueForce=off  PxSenseUpperLimitTorqueForce=off  PxLowerLimitSpecify=off  PxLowerLimitBound=-1  PxLowerLimitBoundUnits=m  PxLowerLimitStiffness=1e6  PxLowerLimitStiffnessUnits=N/m  PxLowerLimitDamping=1e3  PxLowerLimitDampingUnits=N/(m/s)  PxLowerLimitTransitionRegionWidth=1e-4  PxLowerLimitTransitionRegionWidthUnits=m  PxUpperLimitSpecify=off  PxUpperLimitBound=1  PxUpperLimitBoundUnits=m  PxUpperLimitStiffness=1e6  PxUpperLimitStiffnessUnits=N/m  PxUpperLimitDamping=1e3  PxUpperLimitDampingUnits=N/(m/s)  PxUpperLimitTransitionRegionWidth=1e-4  PxUpperLimitTransitionRegionWidthUnits=m  PxPositionTargetSpecify=off  PxPositionTargetPriority=High  PxPositionTargetValue=0  PxPositionTargetValueUnits=m  PxVelocityTargetSpecify=off  PxVelocityTargetPriority=High  PxVelocityTargetValue=0  PxVelocityTargetValueUnits=m/s  PyEquilibriumPosition=0  PyEquilibriumPositionUnits=m  PySpringStiffness=0  PySpringStiffnessUnits=N/m  PyDampingCoefficient=0  PyDampingCoefficientUnits=N/(m/s)  PyTorqueActuationMode=InputTorque  PyMotionActuationMode=ComputedMotion  PySensePosition=off  PySenseVelocity=off  PySenseAcceleration=off  PySenseTorqueForce=off  PySenseLowerLimitTorqueForce=off  PySenseUpperLimitTorqueForce=off  PyLowerLimitSpecify=off  PyLowerLimitBound=-1  PyLowerLimitBoundUnits=m  PyLowerLimitStiffness=1e6  PyLowerLimitStiffnessUnits=N/m  PyLowerLimitDamping=1e3  PyLowerLimitDampingUnits=N/(m/s)  PyLowerLimitTransitionRegionWidth=1e-4  PyLowerLimitTransitionRegionWidthUnits=m  PyUpperLimitSpecify=off  PyUpperLimitBound=1  PyUpperLimitBoundUnits=m  PyUpperLimitStiffness=1e6  PyUpperLimitStiffnessUnits=N/m  PyUpperLimitDamping=1e3  PyUpperLimitDampingUnits=N/(m/s)  PyUpperLimitTransitionRegionWidth=1e-4  PyUpperLimitTransitionRegionWidthUnits=m  PyPositionTargetSpecify=off  PyPositionTargetPriority=High  PyPositionTargetValue=0  PyPositionTargetValueUnits=m  PyVelocityTargetSpecify=off  PyVelocityTargetPriority=High  PyVelocityTargetValue=0  PyVelocityTargetValueUnits=m/s  RzEquilibriumPosition=0  RzEquilibriumPositionUnits=deg  RzSpringStiffness=0  RzSpringStiffnessUnits=N*m/deg  RzDampingCoefficient=0  RzDampingCoefficientUnits=N*m/(deg/s)  RzTorqueActuationMode=NoTorque  RzMotionActuationMode=ComputedMotion  RzSensePosition=off  RzSenseVelocity=off  RzSenseAcceleration=off  RzSenseTorqueForce=off  RzSenseLowerLimitTorqueForce=off  RzSenseUpperLimitTorqueForce=off  RzLowerLimitSpecify=off  RzLowerLimitBound=-90  RzLowerLimitBoundUnits=deg  RzLowerLimitStiffness=1e4  RzLowerLimitStiffnessUnits=N*m/deg  RzLowerLimitDamping=10  RzLowerLimitDampingUnits=N*m/(deg/s)  RzLowerLimitTransitionRegionWidth=0.1  RzLowerLimitTransitionRegionWidthUnits=deg  RzUpperLimitSpecify=off  RzUpperLimitBound=90  RzUpperLimitBoundUnits=deg  RzUpperLimitStiffness=1e4  RzUpperLimitStiffnessUnits=N*m/deg  RzUpperLimitDamping=10  RzUpperLimitDampingUnits=N*m/(deg/s)  RzUpperLimitTransitionRegionWidth=0.1  RzUpperLimitTransitionRegionWidthUnits=deg  RzPositionTargetSpecify=off  RzPositionTargetPriority=High  RzPositionTargetValue=0  RzPositionTargetValueUnits=deg  RzVelocityTargetSpecify=off  RzVelocityTargetPriority=High  RzVelocityTargetValue=0  RzVelocityTargetValueUnits=deg/s
  Simulink-PS Converter : nesl_utility/Simulink-PS Converter  PhysicalDomain=network_engine_domain  SubClassName=ps_input  LeftPortType=input  RightPortType=output  PseudoPeriodic=off  Frequencies=[]  NoiseDistribution=none  NoiseParameters=[]  Unit=1  AffineConversion=off  FilteringAndDerivatives=provide  SimscapeFilterOrder=1  InputFilterTimeConstant=0.001  UdotUserProvided=0
  Simulink-PS Converter1 : nesl_utility/Simulink-PS Converter  PhysicalDomain=network_engine_domain  SubClassName=ps_input  LeftPortType=input  RightPortType=output  PseudoPeriodic=off  Frequencies=[]  NoiseDistribution=none  NoiseParameters=[]  Unit=1  AffineConversion=off  FilteringAndDerivatives=provide  SimscapeFilterOrder=1  InputFilterTimeConstant=0.001  UdotUserProvided=0
  Transform Sensor : sm_lib/Frames and Transforms/Transform Sensor  MeasurementFrame=World  RotationSequence=XYX  SenseAngle=on  SenseAxis=off  SenseQ=off  SenseR=off  SenseRotationSequence=off  SenseOmegaX=off  SenseOmegaY=off  SenseOmegaZ=on  SenseQDot=off  SenseRDot=off  SenseRotationSequenceDot=off  SenseAlphaX=off  SenseAlphaY=off  SenseAlphaZ=off  SenseQDDot=off  SenseRDDot=off  SenseX=on  SenseY=on  SenseZ=off  SenseRad=off  SenseAzim=off  SenseDist=off  SenseInc=off  SenseXDot=on  SenseYDot=on  SenseZDot=off  SenseRadDot=off  SenseAzimDot=off  SenseDistDot=off  SenseIncDot=off  SenseXDDot=off  SenseYDDot=off  SenseZDDot=off  SenseRadDDot=off  SenseAzimDDot=off  SenseDistDDot=off  SenseIncDDot=off
  World Frame : sm_lib/Frames and Transforms/World Frame
  N_Link : PMIOPort  Side=Left
  G : PMIOPort  Port=2  Side=Left
  P_Link : PMIOPort  Port=3  Side=Right
  q1 : PMIOPort  Port=4  Side=Right
  dot q1 : PMIOPort  Port=5  Side=Right
  x1 : PMIOPort  Port=6  Side=Right
  y1 : PMIOPort  Port=7  Side=Right
  vx1 : PMIOPort  Port=8  Side=Right
  vy1 : PMIOPort  Port=9  Side=Right
  wires:
  PS-Simulink Converter2/1 -> Integrator/1
  Constant1/1 -> MATLAB Function/4(cn)
  Constant/1 -> MATLAB Function/3(ct)
  Integrator/1 -> MATLAB Function/5(th)
  PS-Simulink Converter/1 -> MATLAB Function/1(vx)
  PS-Simulink Converter1/1 -> MATLAB Function/2(vy)
  MATLAB Function/2(fy) -> Simulink-PS Converter1/1
  MATLAB Function/1(fx) -> Simulink-PS Converter/1
  connections:
  dot q1/RConn1 -- Transform Sensor/RConn3 -- PS-Simulink Converter2/LConn1
  PS-Simulink Converter1/LConn1 -- Transform Sensor/RConn7 -- vy1/RConn1
  vx1/RConn1 -- Transform Sensor/RConn6 -- PS-Simulink Converter/LConn1
  Transform Sensor/RConn5 -- y1/RConn1
  Transform Sensor/RConn1 -- Brick Solid/RConn1
  x1/RConn1 -- Transform Sensor/RConn4
  P_Link/RConn1 -- Brick Solid/LConn2
  N_Link/RConn1 -- Brick Solid/LConn1
  World Frame/RConn1 -- Transform Sensor/LConn1
  q1/RConn1 -- Transform Sensor/RConn2
  G/RConn1 -- Planar Joint/LConn1
  Simulink-PS Converter1/RConn1 -- Planar Joint/LConn3
  Simulink-PS Converter/RConn1 -- Planar Joint/LConn2
  Brick Solid/RConn2 -- Planar Joint/RConn1

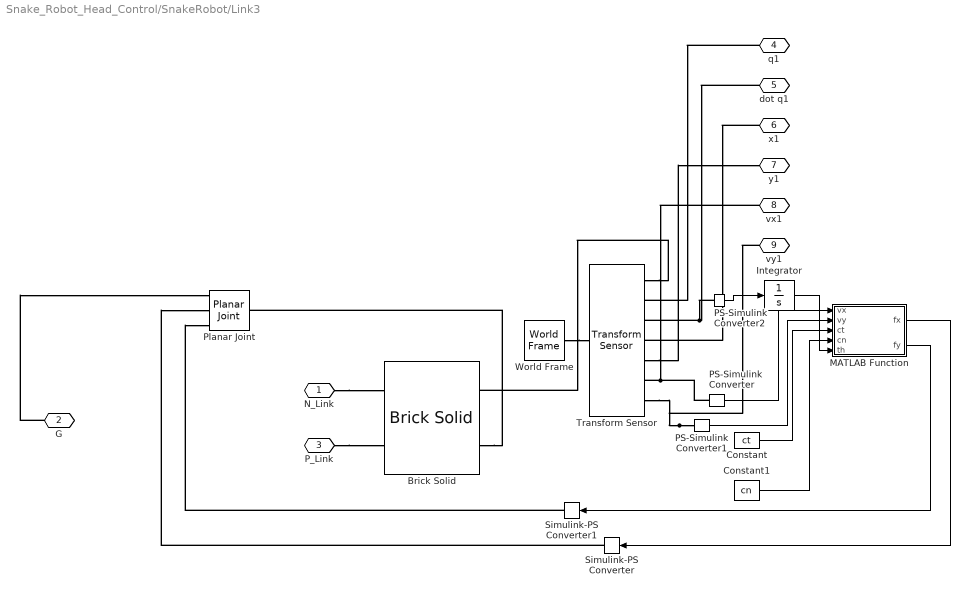
== system Snake_Robot_Head_Control/SnakeRobot/Link3 ==
  Brick Solid : sm_lib/Body Elements/Brick Solid  GraphicAmbientColor=[0.15 0.15 0.15 1.0]  BasedOnType=Mass  BrickDimensions=[180 80 80]  BrickDimensionsUnits=mm  CenterOfMass=[0 0 0]  CenterOfMassUnits=m  GraphicDiffuseColor=[0.5 0.5 0.5]  Density=1000  DensityUnits=kg/m^3  DoExposeReferenceFrame=on  GraphicEmissiveColor=[0.0 0.0 0.0 1.0]  ExportEntireGeometry=off  SerializedFrames=<Frames><Frame><Id>Frame1</Id><Value><Name>nextlink</Name><Origin><Source>GeometricFeature</Source><FeatureName>+x surface</FeatureName></Origin><PrimaryAxis><DefinedDirection>+Z</DefinedDirection><Source>ReferenceFrame</Source><SourceDirection>+Z</SourceDirection><FeatureName></FeatureName></PrimaryAxis><SecondaryAxis><DefinedDirection>+X</DefinedDirection><Source>ReferenceFrame</Source><SourceDirection>+X</SourceDirection><FeatureName></FeatureName></SecondaryAxis></Value></Frame><Frame><Id>Frame2</Id><Value><Name>P_link</Name><Origin><Source>GeometricFeature</Source><FeatureName>-x surface</FeatureName></Origin><PrimaryAxis><DefinedDirection>+Z</DefinedDirection><Source>ReferenceFrame</Source><SourceDirection>+Z</SourceDirection><FeatureName></FeatureName></PrimaryAxis><SecondaryAxis><DefinedDirection>+X</DefinedDirection><Source>ReferenceFrame</Source><SourceDirection>+X</SourceDirection><FeatureName></FeatureName></SecondaryAxis></Value></Frame><Frame><Id>Frame3</Id><Value><Name>F3</Name><Origin><Source>CenterOfMassFrame</Source><FeatureName></FeatureName></Origin><PrimaryAxis><DefinedDirection>+Z</DefinedDirection><Source>ReferenceFrame</Source><SourceDirection>+Z</SourceDirection><FeatureName></FeatureName></PrimaryAxis><SecondaryAxis><DefinedDirection>+X</DefinedDirection><Source>ReferenceFrame</Source><SourceDirection>+X</SourceDirection><FeatureName></FeatureName></SecondaryAxis></Value></Frame></Frames>  MarkerShape=Sphere  MarkerSize=10  GraphicType=FromGeometry  InertiaType=CalculateFromGeometry  Mass=0.9047  MassUnits=kg  MomentsOfInertia=[1 1 1]  MomentsOfInertiaUnits=kg*m^2  GraphicOpacity=1.0  ProductsOfInertia=[0 0 0]  ProductsOfInertiaUnits=kg*m^2  GraphicShininess=75  GraphicSpecularColor=[0.5 0.5 0.5 1.0]  GraphicVisPropType=SimpleVisualProperties
  Constant : Constant  Value=ct
  Constant1 : Constant  Value=cn
  Integrator : Integrator
  MATLAB Function : MATLAB Function  TreatAsAtomicUnit=on
  PS-Simulink Converter : nesl_utility/PS-Simulink Converter  PhysicalDomain=network_engine_domain  SubClassName=ps_output  LeftPortType=input  RightPortType=output  PseudoPeriodic=off  Frequencies=[]  VectorFormat=inherit  Unit=inherit  AffineConversion=off
  PS-Simulink Converter1 : nesl_utility/PS-Simulink Converter  PhysicalDomain=network_engine_domain  SubClassName=ps_output  LeftPortType=input  RightPortType=output  PseudoPeriodic=off  Frequencies=[]  VectorFormat=inherit  Unit=inherit  AffineConversion=off
  PS-Simulink Converter2 : nesl_utility/PS-Simulink Converter  PhysicalDomain=network_engine_domain  SubClassName=ps_output  LeftPortType=input  RightPortType=output  PseudoPeriodic=off  Frequencies=[]  VectorFormat=inherit  Unit=inherit  AffineConversion=off
  Planar Joint : sm_lib/Joints/Planar Joint  JointMode=Normal  SenseConstraintForce=off  SenseConstraintForceX=off  SenseConstraintForceY=off  SenseConstraintForceZ=off  SenseConstraintTorque=off  SenseConstraintTorqueX=off  SenseConstraintTorqueY=off  SenseConstraintTorqueZ=off  SenseTotalForce=off  SenseTotalForceX=off  SenseTotalForceY=off  SenseTotalForceZ=off  SenseTotalTorque=off  SenseTotalTorqueX=off  SenseTotalTorqueY=off  SenseTotalTorqueZ=off  CompositeWrenchDir=FollowerOnBase  CompositeWrenchFrame=BaseFrame  PxEquilibriumPosition=0  PxEquilibriumPositionUnits=m  PxSpringStiffness=0  PxSpringStiffnessUnits=N/m  PxDampingCoefficient=0  PxDampingCoefficientUnits=N/(m/s)  PxTorqueActuationMode=InputTorque  PxMotionActuationMode=ComputedMotion  PxSensePosition=off  PxSenseVelocity=off  PxSenseAcceleration=off  PxSenseTorqueForce=off  PxSenseLowerLimitTorqueForce=off  PxSenseUpperLimitTorqueForce=off  PxLowerLimitSpecify=off  PxLowerLimitBound=-1  PxLowerLimitBoundUnits=m  PxLowerLimitStiffness=1e6  PxLowerLimitStiffnessUnits=N/m  PxLowerLimitDamping=1e3  PxLowerLimitDampingUnits=N/(m/s)  PxLowerLimitTransitionRegionWidth=1e-4  PxLowerLimitTransitionRegionWidthUnits=m  PxUpperLimitSpecify=off  PxUpperLimitBound=1  PxUpperLimitBoundUnits=m  PxUpperLimitStiffness=1e6  PxUpperLimitStiffnessUnits=N/m  PxUpperLimitDamping=1e3  PxUpperLimitDampingUnits=N/(m/s)  PxUpperLimitTransitionRegionWidth=1e-4  PxUpperLimitTransitionRegionWidthUnits=m  PxPositionTargetSpecify=off  PxPositionTargetPriority=High  PxPositionTargetValue=0  PxPositionTargetValueUnits=m  PxVelocityTargetSpecify=off  PxVelocityTargetPriority=High  PxVelocityTargetValue=0  PxVelocityTargetValueUnits=m/s  PyEquilibriumPosition=0  PyEquilibriumPositionUnits=m  PySpringStiffness=0  PySpringStiffnessUnits=N/m  PyDampingCoefficient=0  PyDampingCoefficientUnits=N/(m/s)  PyTorqueActuationMode=InputTorque  PyMotionActuationMode=ComputedMotion  PySensePosition=off  PySenseVelocity=off  PySenseAcceleration=off  PySenseTorqueForce=off  PySenseLowerLimitTorqueForce=off  PySenseUpperLimitTorqueForce=off  PyLowerLimitSpecify=off  PyLowerLimitBound=-1  PyLowerLimitBoundUnits=m  PyLowerLimitStiffness=1e6  PyLowerLimitStiffnessUnits=N/m  PyLowerLimitDamping=1e3  PyLowerLimitDampingUnits=N/(m/s)  PyLowerLimitTransitionRegionWidth=1e-4  PyLowerLimitTransitionRegionWidthUnits=m  PyUpperLimitSpecify=off  PyUpperLimitBound=1  PyUpperLimitBoundUnits=m  PyUpperLimitStiffness=1e6  PyUpperLimitStiffnessUnits=N/m  PyUpperLimitDamping=1e3  PyUpperLimitDampingUnits=N/(m/s)  PyUpperLimitTransitionRegionWidth=1e-4  PyUpperLimitTransitionRegionWidthUnits=m  PyPositionTargetSpecify=off  PyPositionTargetPriority=High  PyPositionTargetValue=0  PyPositionTargetValueUnits=m  PyVelocityTargetSpecify=off  PyVelocityTargetPriority=High  PyVelocityTargetValue=0  PyVelocityTargetValueUnits=m/s  RzEquilibriumPosition=0  RzEquilibriumPositionUnits=deg  RzSpringStiffness=0  RzSpringStiffnessUnits=N*m/deg  RzDampingCoefficient=0  RzDampingCoefficientUnits=N*m/(deg/s)  RzTorqueActuationMode=NoTorque  RzMotionActuationMode=ComputedMotion  RzSensePosition=off  RzSenseVelocity=off  RzSenseAcceleration=off  RzSenseTorqueForce=off  RzSenseLowerLimitTorqueForce=off  RzSenseUpperLimitTorqueForce=off  RzLowerLimitSpecify=off  RzLowerLimitBound=-90  RzLowerLimitBoundUnits=deg  RzLowerLimitStiffness=1e4  RzLowerLimitStiffnessUnits=N*m/deg  RzLowerLimitDamping=10  RzLowerLimitDampingUnits=N*m/(deg/s)  RzLowerLimitTransitionRegionWidth=0.1  RzLowerLimitTransitionRegionWidthUnits=deg  RzUpperLimitSpecify=off  RzUpperLimitBound=90  RzUpperLimitBoundUnits=deg  RzUpperLimitStiffness=1e4  RzUpperLimitStiffnessUnits=N*m/deg  RzUpperLimitDamping=10  RzUpperLimitDampingUnits=N*m/(deg/s)  RzUpperLimitTransitionRegionWidth=0.1  RzUpperLimitTransitionRegionWidthUnits=deg  RzPositionTargetSpecify=off  RzPositionTargetPriority=High  RzPositionTargetValue=0  RzPositionTargetValueUnits=deg  RzVelocityTargetSpecify=off  RzVelocityTargetPriority=High  RzVelocityTargetValue=0  RzVelocityTargetValueUnits=deg/s
  Simulink-PS Converter : nesl_utility/Simulink-PS Converter  PhysicalDomain=network_engine_domain  SubClassName=ps_input  LeftPortType=input  RightPortType=output  PseudoPeriodic=off  Frequencies=[]  NoiseDistribution=none  NoiseParameters=[]  Unit=1  AffineConversion=off  FilteringAndDerivatives=provide  SimscapeFilterOrder=1  InputFilterTimeConstant=0.001  UdotUserProvided=0
  Simulink-PS Converter1 : nesl_utility/Simulink-PS Converter  PhysicalDomain=network_engine_domain  SubClassName=ps_input  LeftPortType=input  RightPortType=output  PseudoPeriodic=off  Frequencies=[]  NoiseDistribution=none  NoiseParameters=[]  Unit=1  AffineConversion=off  FilteringAndDerivatives=provide  SimscapeFilterOrder=1  InputFilterTimeConstant=0.001  UdotUserProvided=0
  Transform Sensor : sm_lib/Frames and Transforms/Transform Sensor  MeasurementFrame=World  RotationSequence=XYX  SenseAngle=on  SenseAxis=off  SenseQ=off  SenseR=off  SenseRotationSequence=off  SenseOmegaX=off  SenseOmegaY=off  SenseOmegaZ=on  SenseQDot=off  SenseRDot=off  SenseRotationSequenceDot=off  SenseAlphaX=off  SenseAlphaY=off  SenseAlphaZ=off  SenseQDDot=off  SenseRDDot=off  SenseX=on  SenseY=on  SenseZ=off  SenseRad=off  SenseAzim=off  SenseDist=off  SenseInc=off  SenseXDot=on  SenseYDot=on  SenseZDot=off  SenseRadDot=off  SenseAzimDot=off  SenseDistDot=off  SenseIncDot=off  SenseXDDot=off  SenseYDDot=off  SenseZDDot=off  SenseRadDDot=off  SenseAzimDDot=off  SenseDistDDot=off  SenseIncDDot=off
  World Frame : sm_lib/Frames and Transforms/World Frame
  N_Link : PMIOPort  Side=Left
  G : PMIOPort  Port=2  Side=Left
  P_Link : PMIOPort  Port=3  Side=Right
  q1 : PMIOPort  Port=4  Side=Right
  dot q1 : PMIOPort  Port=5  Side=Right
  x1 : PMIOPort  Port=6  Side=Right
  y1 : PMIOPort  Port=7  Side=Right
  vx1 : PMIOPort  Port=8  Side=Right
  vy1 : PMIOPort  Port=9  Side=Right
  wires:
  PS-Simulink Converter2/1 -> Integrator/1
  Constant1/1 -> MATLAB Function/4(cn)
  Constant/1 -> MATLAB Function/3(ct)
  Integrator/1 -> MATLAB Function/5(th)
  PS-Simulink Converter/1 -> MATLAB Function/1(vx)
  PS-Simulink Converter1/1 -> MATLAB Function/2(vy)
  MATLAB Function/2(fy) -> Simulink-PS Converter1/1
  MATLAB Function/1(fx) -> Simulink-PS Converter/1
  connections:
  dot q1/RConn1 -- Transform Sensor/RConn3 -- PS-Simulink Converter2/LConn1
  PS-Simulink Converter1/LConn1 -- Transform Sensor/RConn7 -- vy1/RConn1
  vx1/RConn1 -- Transform Sensor/RConn6 -- PS-Simulink Converter/LConn1
  Transform Sensor/RConn5 -- y1/RConn1
  Transform Sensor/RConn1 -- Brick Solid/RConn1
  x1/RConn1 -- Transform Sensor/RConn4
  P_Link/RConn1 -- Brick Solid/LConn2
  N_Link/RConn1 -- Brick Solid/LConn1
  World Frame/RConn1 -- Transform Sensor/LConn1
  q1/RConn1 -- Transform Sensor/RConn2
  G/RConn1 -- Planar Joint/LConn1
  Simulink-PS Converter1/RConn1 -- Planar Joint/LConn3
  Simulink-PS Converter/RConn1 -- Planar Joint/LConn2
  Brick Solid/RConn2 -- Planar Joint/RConn1
